simulink model "Bat_EQC"  (R2024a)
settings: Solver=FixedStepAuto  StartTime=0.0  StopTime=t_end  FixedStep=dt  MaxStep=Ts  RelTol=1e-3  EnableMultiTasking=on
values from neighbouring files (symbols this model uses):
  I = squeeze(out.I.Data)./4.6    [PI_init.m]
  P0 = 4.1374e3    (= 4137.4)    [PI_init.m]
  P_crit = 158e3    (= 158000)    [PI_init.m]
  Parameters = [Q,Rs,Rbat1,Cbat1,alpha,beta,Tamb,h,A_surf,kb,E_SEI,A_SEI,m_cell,Cp,m_an,h_SEI]    [PI_init.m]
  Params_P = [sig0,P_atm,E,alpha_cell,Tamb,L,Vh0,A_surf,m_an,xSEI0,MC6,R,A1,B1,     C1,A2,B2,C2,yEC,yDMC]    [PI_init.m]
  Tmax = 80+273.15    (= 353.15)    [PI_init.m]
  V_min = 0    [PI_init.m]
  xi_init = [1,0,Tamb,xSEI0]'    [PI_init.m]
libraries: slpidlib x2
settings Model: Creator=imanebrahimi  LastModifiedBy=imanebrahimi
settings SolverCC: AutoInsertRateTranBlk=on
settings OptimizationCC: DefaultParameterBehavior=Inlined  InlineInvariantSignals=on  EnhancedBackFolding=on  PassReuseOutputArgsAs=Individual arguments  StateBitsets=on  DataBitsets=on  ZeroExternalMemoryAtStartup=off  ZeroInternalMemoryAtStartup=off  NoFixptDivByZeroProtection=on  LifeSpan=1  OptimizeBlockOrder=speed  DifferentSizesBufferReuse=on  EfficientTunableParamExpr=on
settings DebuggingCC: ParameterTunabilityLossMsg=error
settings HardwareCC: ProdBitPerPointer=32  ProdBitPerSizeT=32  ProdBitPerPtrDiffT=32  ProdLargestAtomicFloat=None  ProdIntDivRoundTo=Floor  ProdWordSize=32  ProdHWDeviceType=Generic->Custom
settings SFSimCC: MATLABDynamicMemAlloc=off
settings RTWCC: Description=Embedded Coder  SystemTargetFile=ert.tlc  TLCOptions=-p0  GenCodeOnly=on  TemplateMakefile=ert_default_tmf  GenerateReport=on  RTWVerbose=off  IncludeHyperlinkInReport=on  LaunchReport=on  GPUComputeCapability=3.5
settings CodeAppCC: ForceParamTrailComments=on  IgnoreCustomStorageClasses=off  OperatorAnnotations=on  SimulinkDataObjDesc=on  SFDataObjDesc=on  CustomSymbolStrGlobalVar=rt$N$M  CustomSymbolStrType=$N$M  CustomSymbolStrFcn=$N$M$F  CustomSymbolStrMacro=$N$M  InsertBlockDesc=on
settings ERTTargetCC: TargetLangStandard=C99 (ISO)  CodeReplacementLibrary=ISO_C  GenerateSampleERTMain=on  IncludeMdlTerminateFcn=off  SuppressErrorStatus=on  SupportAbsoluteTime=off  PurelyIntegerCode=on  SupportNonFinite=off  SupportComplex=off  InlinedParameterPlacement=NonHierarchical  RootIOFormat=Structure reference  ERTCustomFileTemplate=example_file_process.tlc

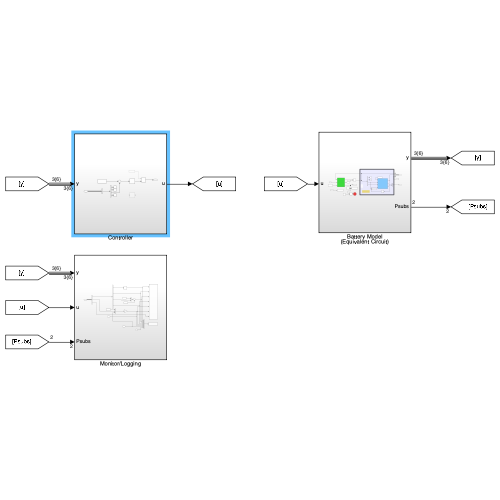
[thumbnail: Simulink's stored preview of the top-level diagram]
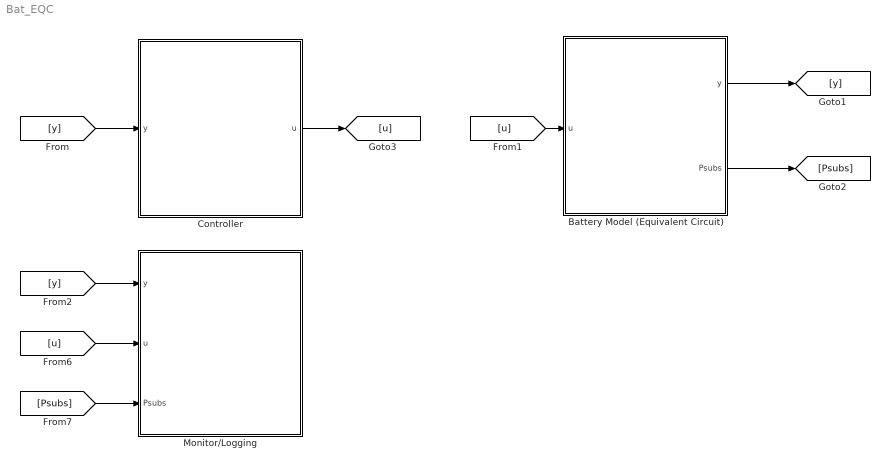
== system Bat_EQC ==
  Battery Model (Equivalent Circuit) : Subsystem
  Controller : Subsystem
  Monitor/Logging : Subsystem
  wires:
  [u] -> Monitor/Logging/2(u)
  [Psubs] -> Monitor/Logging/3(Psubs)
  Battery Model (Equivalent Circuit)/1(y) -> [y]
  Battery Model (Equivalent Circuit)/2(Psubs) -> [Psubs]
  [u] -> Battery Model (Equivalent Circuit)/1(u)
  [y] -> Monitor/Logging/1(y)
  [y] -> Controller/1(y)
  Controller/1(u) -> [u]

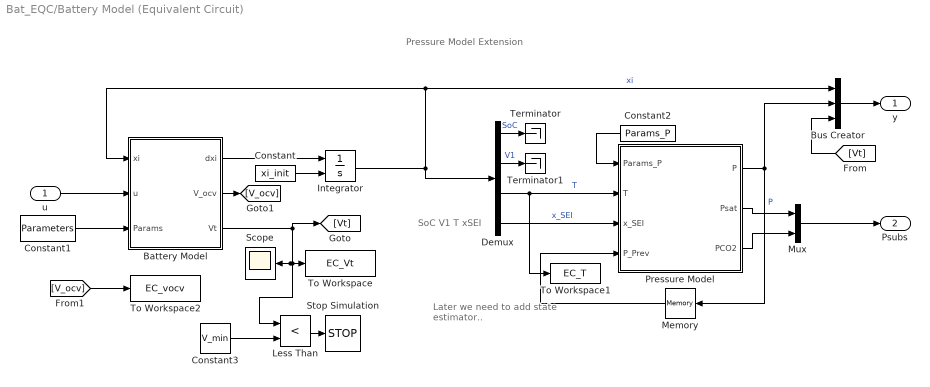
== system Bat_EQC/Battery Model (Equivalent Circuit) ==
  note: Pressure Model Extension
  note: Later we need to add state estimator..
  note: SoC
      | V1
      | T
      | xSEI
  u : Inport
  Battery Model : MATLAB Function  TreatAsAtomicUnit=on
  Bus Creator : BusCreator  Inputs=3
  Constant : Constant  Value=xi_init
  Constant1 : Constant  Value=Parameters
  Constant2 : Constant  Value=Params_P
  Constant3 : Constant  Value=V_min
  Demux : Demux
  Integrator : Integrator  InitialConditionSource=external
  Less Than : RelationalOperator  Operator=<  OutDataTypeStr=boolean  RndMeth=Simplest  InputSameDT=off
  Memory : Memory  InitialCondition=P0  InheritSampleTime=on  LinearizeAsDelay=on
  Mux : Mux  Inputs=2
  Pressure Model : MATLAB Function  TreatAsAtomicUnit=on
  Scope : Scope
  Stop Simulation : Stop
  Terminator : Terminator
  Terminator1 : Terminator
  To Workspace : ToWorkspace  VariableName=EC_Vt  SaveFormat=Timeseries  SampleTime=-1
  To Workspace1 : ToWorkspace  VariableName=EC_T  SaveFormat=Timeseries  SampleTime=-1
  To Workspace2 : ToWorkspace  VariableName=EC_vocv  SaveFormat=Timeseries  SampleTime=-1
  y : Outport
  Psubs : Outport  Port=2
  wires:
  u/1 -> Battery Model/2(u)
  Battery Model/1(dxi) -> Integrator/1
  Constant/1 -> Integrator/2
  Integrator/1 -> Demux/1, Bus Creator/1, Battery Model/1(xi)  "xi"
  Constant1/1 -> Battery Model/3(Params)
  Demux/2 -> Terminator1/1  "V1"
  Demux/3 -> To Workspace1/1, Pressure Model/2(T)  "T"
  Demux/4 -> Pressure Model/3(x_SEI)  "x_SEI"
  Demux/1 -> Terminator/1  "SoC"
  Pressure Model/1(P) -> Memory/1, Bus Creator/2  "P"
  Memory/1 -> Pressure Model/4(P_Prev)
  Constant2/1 -> Pressure Model/1(Params_P)
  Bus Creator/1 -> y/1
  Pressure Model/3(PCO2) -> Mux/2
  Pressure Model/2(Psat) -> Mux/1
  Mux/1 -> Psubs/1
  Battery Model/3(Vt) -> [Vt], To Workspace/1, Scope/1, Less Than/1
  Constant3/1 -> Less Than/2
  Less Than/1 -> Stop Simulation/1
  [Vt] -> Bus Creator/3
  Battery Model/2(V_ocv) -> [V_ocv]
  [V_ocv] -> To Workspace2/1

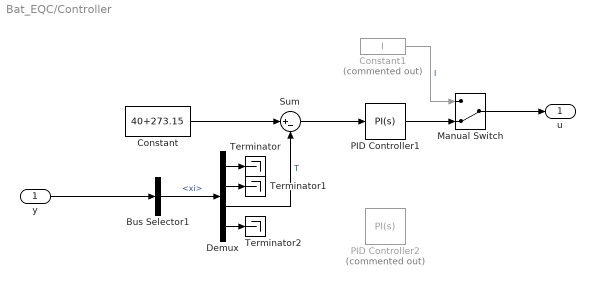
== system Bat_EQC/Controller ==
  y : Inport
  Bus Selector1 : BusSelector  OutputSignals=xi
  Constant : Constant  Value=40+273.15
  Constant1 : Constant  Commented=on  Value=I
  Demux : Demux
  Manual Switch : ManualSwitch  CurrentSetting=0
  PID Controller1 : slpidlib/PID Controller  Controller=PI  Form=Parallel  TimeDomain=Continuous-time  UseExternalTs=off  SampleTime=-1  IntegratorMethod=Forward Euler  FilterMethod=Forward Euler  ControllerParametersSource=internal  P=7.95363343093835  I=0.0486588718627495  UseKiTs=off  D=0  UseExternalDerivativeSource=off  N=100  UseFilter=on  TunerSelectOption=Transfer Function Based (PID Tuner App)  InitialConditionSource=internal  InitialConditionForIntegrator=0  InitialConditionForFilter=0  DifferentiatorICPrevScaledInput=0  ExternalReset=none  TrackingMode=off  Kt=1  LimitOutput=off  SatLimitsSource=internal  UpperSaturationLimit=46  LowerSaturationLimit=0  LinearizeAsGain=on  AntiWindupMode=none  Kb=1  LimitIntegrator=off  UpperIntegratorSaturationLimit=inf  LowerIntegratorSaturationLimit=-inf  POutMin=[]  POutMax=[]  IOutMin=[]  IOutMax=[]  DOutMin=[]  DOutMax=[]  NOutMin=[]  NOutMax=[]  SumOutMin=[]  SumOutMax=[]  SaturationOutMin=[]  SaturationOutMax=[]  PParamMin=[]  PParamMax=[]  IParamMin=[]  IParamMax=[]  DParamMin=[]  DParamMax=[]  NParamMin=[]  NParamMax=[]  KbParamMin=[]  KbParamMax=[]  KtParamMin=[]  KtParamMax=[]  KbOutMin=[]  KbOutMax=[]  KtOutMin=[]  KtOutMax=[]  IntegratorOutMin=[]  IntegratorOutMax=[]  FilterOutMin=[]  FilterOutMax=[]  SumI1OutMin=[]  SumI1OutMax=[]  SumI2OutMin=[]  SumI2OutMax=[]  SumI3OutMin=[]  SumI3OutMax=[]  SumI4OutMin=[]  SumI4OutMax=[]  SumDOutMin=[]  SumDOutMax=[]  DifferentiatorOutMin=[]  DifferentiatorOutMax=[]  FilterDiffOutCoefMin=[]  FilterDiffOutCoefMax=[]  ReciprocalOutMin=[]  ReciprocalOutMax=[]  SumDenOutMin=[]  SumDenOutMax=[]  SumNumOutMin=[]  SumNumOutMax=[]  DivideOutMin=[]  DivideOutMax=[]  UdiffTsProdOutMin=[]  UdiffTsProdOutMax=[]  NTsProdOutMin=[]  NTsProdOutMax=[]  UintegralTsProdOutMin=[]  UintegralTsProdOutMax=[]  UngainTsProdOutMin=[]  UngainTsProdOutMax=[]  ClampingZeroOutDataTypeStr=Inherit: Inherit via back propagation  ClampingZeroOutMin=[]  ClampingZeroOutMax=[]  FilterDenConstantOutDataTypeStr=Inherit: Inherit via back propagation  FilterDenConstantOutMin=[]  FilterDenConstantOutMax=[]  PCopyOutDataTypeStr=Inherit: Inherit via back propagation  PCopyOutMin=[]  PCopyOutMax=[]  NCopyOutDataTypeStr=Inherit: Inherit via back propagation  NCopyOutMin=[]  NCopyOutMax=[]  IntegratorContinuousStateAttributes=''  IntegratorStateMustResolveToSignalObject=off  IntegratorRTWStateStorageClass=Auto  FilterContinuousStateAttributes=''  FilterStateMustResolveToSignalObject=off  FilterRTWStateStorageClass=Auto  ParallelPVariant=InternalParameters  IdealPVariant=Disabled  IVariant=InternalParameters  DVariant=Disabled  IntegratorVariant=Continuous  SatVariant=Disabled  AWVariant=Passthrough  PCopyVariant=Disabled  TRVariant=Disabled  FdbkBlocksVariant=Forward  IdealPFdbkVariant=Disabled  SatFdbkVariant=Disabled  DerivativeFilterVariant=Disabled  NVariant=Disabled  NCopyVariant=Disabled_SignalSpec  FilterICVariant=Disabled  IntegratorICVariant=InternalICs  ExternalResetVariant=Disabled  TRSumVariant=Passthrough  SumFdbkVariant=Disabled  SumVariant=Sum_PI  TsampFilterVariant=InternalTs  TsampNgainVariant=Passthrough  TsampIntegralVariant=Disabled_SignalSpec  ExternalSaturationOutDataTypeStr=Inherit: Same as second input  DerivativeSourceVariant=Disabled
  PID Controller2 : slpidlib/PID Controller  Commented=on  Controller=PI  Form=Parallel  TimeDomain=Continuous-time  UseExternalTs=off  SampleTime=-1  IntegratorMethod=Forward Euler  FilterMethod=Forward Euler  ControllerParametersSource=internal  P=0.0899141239627344  I=8.03567670812028e-05  UseKiTs=off  D=0  UseExternalDerivativeSource=off  N=100  UseFilter=on  TunerSelectOption=Transfer Function Based (PID Tuner App)  InitialConditionSource=internal  InitialConditionForIntegrator=0  InitialConditionForFilter=0  DifferentiatorICPrevScaledInput=0  ExternalReset=none  TrackingMode=off  Kt=1  LimitOutput=on  SatLimitsSource=internal  UpperSaturationLimit=46  LowerSaturationLimit=0  LinearizeAsGain=on  AntiWindupMode=none  Kb=1  LimitIntegrator=off  UpperIntegratorSaturationLimit=inf  LowerIntegratorSaturationLimit=-inf  POutMin=[]  POutMax=[]  IOutMin=[]  IOutMax=[]  DOutMin=[]  DOutMax=[]  NOutMin=[]  NOutMax=[]  SumOutMin=[]  SumOutMax=[]  SaturationOutMin=[]  SaturationOutMax=[]  PParamMin=[]  PParamMax=[]  IParamMin=[]  IParamMax=[]  DParamMin=[]  DParamMax=[]  NParamMin=[]  NParamMax=[]  KbParamMin=[]  KbParamMax=[]  KtParamMin=[]  KtParamMax=[]  KbOutMin=[]  KbOutMax=[]  KtOutMin=[]  KtOutMax=[]  IntegratorOutMin=[]  IntegratorOutMax=[]  FilterOutMin=[]  FilterOutMax=[]  SumI1OutMin=[]  SumI1OutMax=[]  SumI2OutMin=[]  SumI2OutMax=[]  SumI3OutMin=[]  SumI3OutMax=[]  SumI4OutMin=[]  SumI4OutMax=[]  SumDOutMin=[]  SumDOutMax=[]  DifferentiatorOutMin=[]  DifferentiatorOutMax=[]  FilterDiffOutCoefMin=[]  FilterDiffOutCoefMax=[]  ReciprocalOutMin=[]  ReciprocalOutMax=[]  SumDenOutMin=[]  SumDenOutMax=[]  SumNumOutMin=[]  SumNumOutMax=[]  DivideOutMin=[]  DivideOutMax=[]  UdiffTsProdOutMin=[]  UdiffTsProdOutMax=[]  NTsProdOutMin=[]  NTsProdOutMax=[]  UintegralTsProdOutMin=[]  UintegralTsProdOutMax=[]  UngainTsProdOutMin=[]  UngainTsProdOutMax=[]  ClampingZeroOutDataTypeStr=Inherit: Inherit via back propagation  ClampingZeroOutMin=[]  ClampingZeroOutMax=[]  FilterDenConstantOutDataTypeStr=Inherit: Inherit via back propagation  FilterDenConstantOutMin=[]  FilterDenConstantOutMax=[]  PCopyOutDataTypeStr=Inherit: Inherit via back propagation  PCopyOutMin=[]  PCopyOutMax=[]  NCopyOutDataTypeStr=Inherit: Inherit via back propagation  NCopyOutMin=[]  NCopyOutMax=[]  IntegratorContinuousStateAttributes=''  IntegratorStateMustResolveToSignalObject=off  IntegratorRTWStateStorageClass=Auto  FilterContinuousStateAttributes=''  FilterStateMustResolveToSignalObject=off  FilterRTWStateStorageClass=Auto  ParallelPVariant=InternalParameters  IdealPVariant=Disabled  IVariant=InternalParameters  DVariant=Disabled  IntegratorVariant=Continuous  SatVariant=Enabled  AWVariant=Passthrough  PCopyVariant=Disabled  TRVariant=Disabled  FdbkBlocksVariant=Forward  IdealPFdbkVariant=Disabled  SatFdbkVariant=Disabled  DerivativeFilterVariant=Disabled  NVariant=Disabled  NCopyVariant=Disabled_SignalSpec  FilterICVariant=Disabled  IntegratorICVariant=InternalICs  ExternalResetVariant=Disabled  TRSumVariant=Passthrough  SumFdbkVariant=Disabled  SumVariant=Sum_PI  TsampFilterVariant=InternalTs  TsampNgainVariant=Passthrough  TsampIntegralVariant=Disabled_SignalSpec  ExternalSaturationOutDataTypeStr=Inherit: Same as second input  DerivativeSourceVariant=Disabled
  Sum : Sum  Inputs=|+-
  Terminator : Terminator
  Terminator1 : Terminator
  Terminator2 : Terminator
  u : Outport
  wires:
  Manual Switch/1 -> u/1
  Sum/1 -> PID Controller1/1
  PID Controller1/1 -> Manual Switch/2
  y/1 -> Bus Selector1/1
  Demux/4 -> Terminator2/1
  Demux/1 -> Terminator/1
  Demux/2 -> Terminator1/1
  Bus Selector1/1 -> Demux/1  "<xi>"
  Demux/3 -> Sum/2  "T"
  Constant/1 -> Sum/1
  Constant1/1 -> Manual Switch/1  "I"

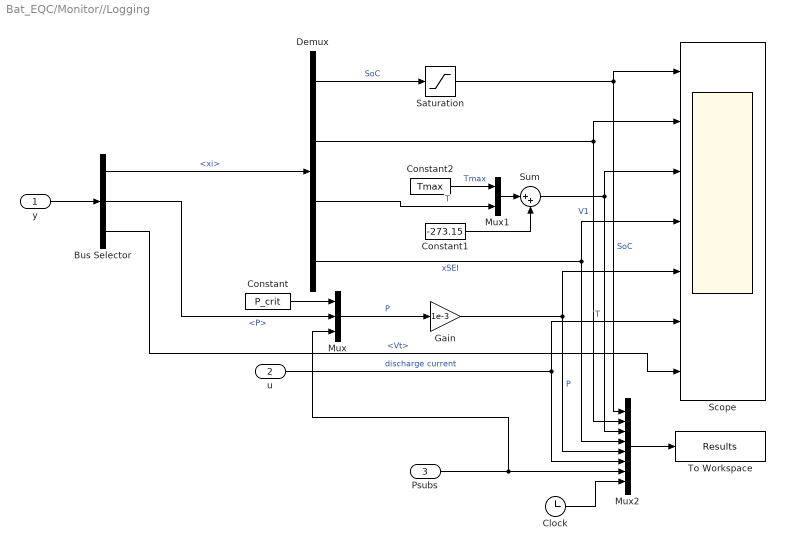
== system Bat_EQC/Monitor//Logging ==
  y : Inport
  u : Inport  Port=2
  Psubs : Inport  Port=3
  Bus Selector : BusSelector  OutputSignals=xi,P,Vt
  Clock : Clock
  Constant : Constant  Value=P_crit
  Constant1 : Constant  Value=-273.15
  Constant2 : Constant  Value=Tmax
  Demux : Demux
  Gain : Gain  Gain=1e-3
  Mux : Mux  Inputs=3
  Mux1 : Mux  Inputs=2
  Mux2 : Mux  Inputs=8
  Saturation : Saturate  UpperLimit=1  LowerLimit=0
  Scope : Scope  NumInputPorts=7
  Sum : Sum  Inputs=|++
  To Workspace : ToWorkspace  VariableName=Results  SampleTime=-1
  wires:
  Demux/1 -> Saturation/1  "SoC"
  Saturation/1 -> Scope/1, Mux2/1  "SoC"
  Constant1/1 -> Sum/2
  Demux/4 -> Mux2/4, Scope/4  "xSEI"
  Demux/2 -> Scope/2, Mux2/2  "V1"
  Constant/1 -> Mux/1
  Mux/1 -> Gain/1  "P"
  Sum/1 -> Mux2/3, Scope/3  "T"
  Constant2/1 -> Mux1/1  "Tmax"
  Mux1/1 -> Sum/1
  Demux/3 -> Mux1/2  "T"
  Gain/1 -> Mux2/5, Scope/5  "P"
  u/1 -> Mux2/6, Scope/6  "discharge current"
  Mux2/1 -> To Workspace/1
  Clock/1 -> Mux2/8
  Psubs/1 -> Mux/3, Mux2/7
  Bus Selector/2 -> Mux/2  "<P>"
  y/1 -> Bus Selector/1
  Bus Selector/3 -> Scope/7  "<Vt>"
  Bus Selector/1 -> Demux/1  "<xi>"

== matlab function Bat_EQC/Battery Model (Equivalent Circuit)/Battery Model ==
  data: xi input; dxi output; V_ocv output; u input; Params input; Vt output
% Script by: Iman Ebrahimi (iebrahimi@ucmerced.edu) - CastroLab UC Merced
function [dxi,V_ocv,Vt]  = Battery(xi,u,Params) 
%% Parameters
Q       = Params(1);
Rs      = Params(2);
R1      = Params(3);
C1      = Params(4);
alpha   = Params(5);
beta    = Params(6);
Tamb    = Params(7);
h       = Params(8);
A_surf  = Params(9); 
kb      = Params(10);
E_SEI   = Params(11);
A_SEI   = Params(12);
m_cell  = Params(13);
Cp      = Params(14);
m_an    = Params(15);
h_SEI   = Params(16);

%% Inputs
I       = u;
%% States
SoC     = xi(1);
if SoC<=0
    SoC = 0;
else
    SoC = xi(1);
end

V1      = xi(2);
T       = xi(3);
xSEI    = xi(4);

%% Evolution of the states
dxi     = zeros(4,1);
% Equations
dxi(1)  = -I/Q;
dxi(2)  = -V1/(alpha*R1*beta*C1)+I/(beta*C1);
Q_ohm   = I^2*Rs+I*V1; 
Q_SEI   = -m_an*h_SEI*(-A_SEI*xSEI*exp(-E_SEI/(kb*T)));
dxi(3)  = (Q_ohm+Q_SEI-h*A_surf*(T-Tamb))/(m_cell*Cp); % Q_SEI is neglected here
dxi(4)  = -A_SEI*xSEI*exp(-E_SEI/(kb*T));

V_ocv   = [0.114319142120841  -0.663997904709863 ...
            1.686768366470837  -2.462409468590447   2.282769243949050 ...
            -1.401600551327618   0.576551904459066  -0.157044814050174 ...
            0.027351974716897  -0.002866912229499   0.000171009483610...
            0.000029999998915].*1e5*SoC.^(11:-1:0)';
Rss     = 0.0048*exp(31.0494/(298-(-15.3253)));
Vt      = V_ocv-Rss*I-V1;

== matlab function Bat_EQC/Battery Model (Equivalent Circuit)/Pressure Model ==
  data: Params_P input; T input; x_SEI input; P_Prev input; P output; Psat output; PCO2 output
function [P,Psat,PCO2] = Pressure(Params_P,T,x_SEI,P_Prev)

% Parameters
sig0        = Params_P(1);
P_atm       = Params_P(2);
E           = Params_P(3);
alpha_cell  = Params_P(4);
Tamb        = Params_P(5);
L           = Params_P(6);
Vh0         = Params_P(7);
A_surf      = Params_P(8);
m_an        = Params_P(9);
xSEI0       = Params_P(10);
MC6         = Params_P(11);
R           = Params_P(12);
A1          = Params_P(13);
B1          = Params_P(14);
C1          = Params_P(15);
A2          = Params_P(16);
B2          = Params_P(17);
C2          = Params_P(18);
yEC         = Params_P(19);
yDMC        = Params_P(20);

% Pressure (Algebraic) model
d_sigma     = max(P_Prev-sig0-P_atm,E*alpha_cell*(T-Tamb)/L);
dd          = L*d_sigma/E;
Vh          = Vh0+A_surf*(dd-alpha_cell*(T-Tamb));
nCO2        = m_an*(xSEI0-x_SEI)/(2*MC6);                        % [mol]
PCO2        = nCO2*R*T/Vh;                                       % [Pa]
PsatEC      = (10^(A1-B1/(T+C1)))*1e3;                           % [Pa]
PsatDMC     = (10^(A2-B2/(T+C2)))*1e3;                           % [Pa]
Psat        = yEC*PsatEC+yDMC*PsatDMC;                           % [Pa]
P           = PCO2+Psat;                                         % [Pa]
